simulink model "simu"  (R2024a)
settings: Solver=VariableStepAuto  StartTime=0.0  StopTime=10.0  RelTol=1e-3
settings Model: Creator=a2152355  LastModifiedBy=a2152355

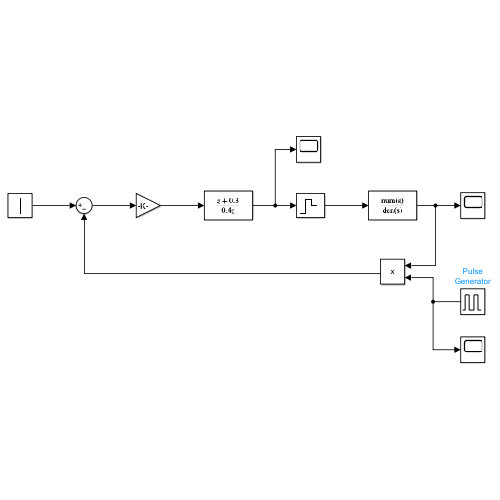
[thumbnail: Simulink's stored preview of the top-level diagram]
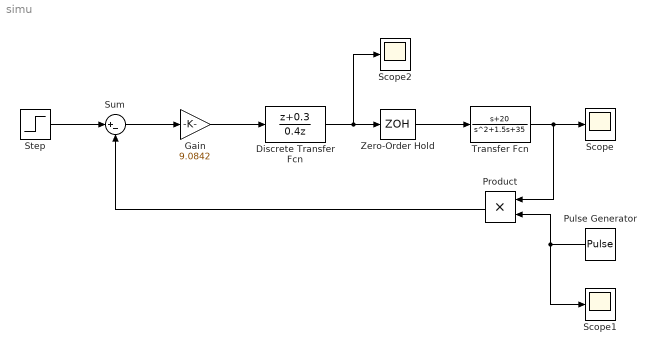
== system simu ==
  Discrete Transfer Fcn : DiscreteTransferFcn  Numerator=[1 0.3]  Denominator=[0.4 0]
  Gain : Gain  Gain=9.0842
  Product : Product
  Pulse Generator : DiscretePulseGenerator  PulseType=Time based  Period=10  PulseWidth=5
  Scope : Scope
  Scope1 : Scope
  Scope2 : Scope
  Step : Step  SampleTime=0
  Sum : Sum  Inputs=|+-
  Transfer Fcn : TransferFcn  Numerator=[1 20]  Denominator=[1 1.5 35]
  Zero-Order Hold : ZeroOrderHold  SampleTime=-1
  wires:
  Step/1 -> Sum/1
  Sum/1 -> Gain/1
  Product/1 -> Sum/2
  Discrete Transfer Fcn/1 -> Scope2/1, Zero-Order Hold/1
  Gain/1 -> Discrete Transfer Fcn/1
  Zero-Order Hold/1 -> Transfer Fcn/1
  Transfer Fcn/1 -> Product/1, Scope/1
  Pulse Generator/1 -> Product/2, Scope1/1
